simulink model "chapter2"  (R2020b)
settings: Solver=ode4  StartTime=0.0  StopTime=5  FixedStep=0.001  RelTol=1e-3
settings Model: Creator=yuto  LastModifiedBy=yuto
settings DataIOCC: ReturnWorkspaceOutputs=off

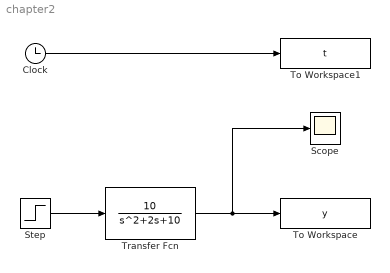
== system chapter2 ==
  Clock : Clock
  Scope : Scope
  Step : Step  SampleTime=0
  To Workspace : ToWorkspace  VariableName=y  SampleTime=-1
  To Workspace1 : ToWorkspace  VariableName=t  SampleTime=-1
  Transfer Fcn : TransferFcn  Numerator=[10]  Denominator=[1 2 10]
  wires:
  Step/1 -> Transfer Fcn/1
  Transfer Fcn/1 -> Scope/1, To Workspace/1
  Clock/1 -> To Workspace1/1
